simulink model "model_crmorm"  (R2012b)
settings: Solver=ode45  StartTime=0.0  StopTime=tsim  MaxStep=0.01  RelTol=1e-3
values from neighbouring files (symbols this model uses):
  am = -1    [master_crmorm.m]
  ap = 1    [master_crmorm.m]
  gamma = 100    [sim_setup.m]
  km = 1    [master_crmorm.m]
  kp = 2    [master_crmorm.m]
  l = -1000    [sim_setup.m]
  xp0 = 0    [master_crmorm.m]
settings Model: Creator=Dan  LastModifiedBy=Dan

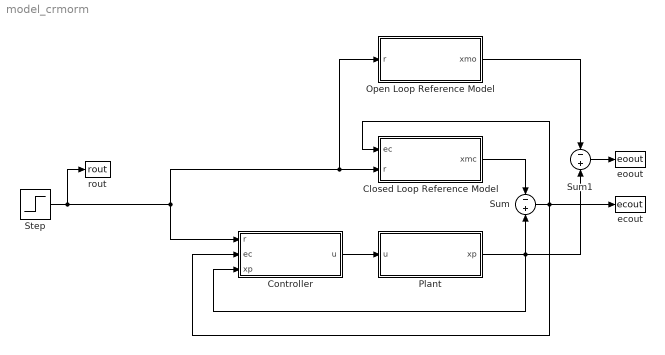
== system model_crmorm ==
  Closed Loop Reference Model : Subsystem
  Controller : Subsystem
  Open Loop Reference Model : Subsystem
  Plant : Subsystem
  Step : Step  Time=5  SampleTime=0
  Sum : Sum  Inputs=-|+
  Sum1 : Sum  Inputs=-|+
  ecout : ToWorkspace  VariableName=ecout  SampleTime=-1  SaveFormat=Structure With Time
  eoout : ToWorkspace  VariableName=eoout  SampleTime=-1  SaveFormat=Structure With Time
  rout : ToWorkspace  VariableName=rout  SampleTime=-1  SaveFormat=Structure With Time
  wires:
  Step/1 -> rout/1, Open Loop Reference Model/1(r), Closed Loop Reference Model/2(r), Controller/1(r)
  Controller/1(u) -> Plant/1(u)
  Plant/1(xp) -> Sum1/2, Sum/2, Controller/3(xp)
  Closed Loop Reference Model/1(xmc) -> Sum/1
  Sum/1 -> ecout/1, Controller/2(ec), Closed Loop Reference Model/1(ec)
  Open Loop Reference Model/1(xmo) -> Sum1/1
  Sum1/1 -> eoout/1

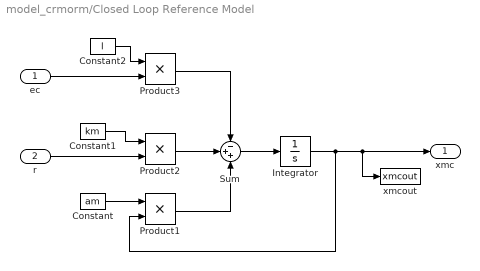
== system model_crmorm/Closed Loop Reference Model ==
  ec : Inport
  r : Inport  Port=2
  Constant : Constant  Value=am
  Constant1 : Constant  Value=km
  Constant2 : Constant  Value=l
  Integrator : Integrator
  Product1 : Product  RndMeth=Zero
  Product2 : Product  RndMeth=Zero
  Product3 : Product  RndMeth=Zero
  Sum : Sum  Inputs=-++
  xmcout : ToWorkspace  VariableName=xmcout  SampleTime=-1  SaveFormat=Structure With Time
  xmc : Outport
  wires:
  Constant/1 -> Product1/1
  Integrator/1 -> xmcout/1, xmc/1, Product1/2
  Constant1/1 -> Product2/1
  Sum/1 -> Integrator/1
  r/1 -> Product2/2
  ec/1 -> Product3/2
  Constant2/1 -> Product3/1
  Product2/1 -> Sum/2
  Product1/1 -> Sum/3
  Product3/1 -> Sum/1

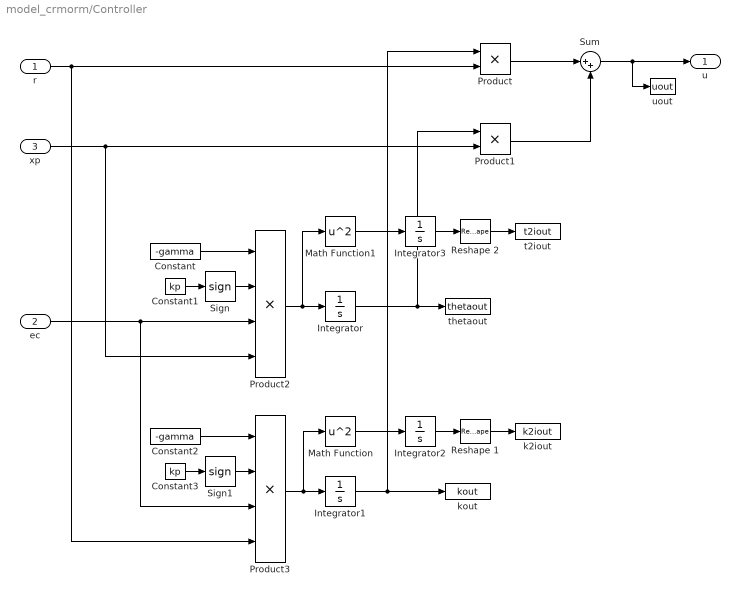
== system model_crmorm/Controller ==
  r : Inport
  ec : Inport  Port=2
  xp : Inport  Port=3
  Constant : Constant  Value=-gamma
  Constant1 : Constant  Value=kp
  Constant2 : Constant  Value=-gamma
  Constant3 : Constant  Value=kp
  Integrator{,1..3} (4 alike) : Integrator
  Math Function : Math  Operator=square  SaturateOnIntegerOverflow=on
  Math Function1 : Math  Operator=square  SaturateOnIntegerOverflow=on
  Product : Product  RndMeth=Zero
  Product1 : Product  RndMeth=Zero
  Product2 : Product  Inputs=4  RndMeth=Zero
  Product3 : Product  Inputs=4  RndMeth=Zero
  Reshape 1 : Reshape
  Reshape 2 : Reshape
  Sign : Signum
  Sign1 : Signum
  Sum : Sum  Inputs=|++
  k2iout : ToWorkspace  VariableName=k2iout  SampleTime=-1  SaveFormat=Structure With Time
  kout : ToWorkspace  VariableName=kout  SampleTime=-1  SaveFormat=Structure With Time
  t2iout : ToWorkspace  VariableName=t2iout  SampleTime=-1  SaveFormat=Structure With Time
  thetaout : ToWorkspace  VariableName=thetaout  SampleTime=-1  SaveFormat=Structure With Time
  uout : ToWorkspace  VariableName=uout  SampleTime=-1  SaveFormat=Structure With Time
  u : Outport
  wires:
  Product/1 -> Sum/1
  Product1/1 -> Sum/2
  r/1 -> Product3/4, Product/2
  xp/1 -> Product2/4, Product1/2
  Sum/1 -> uout/1, u/1
  Constant/1 -> Product2/1
  Sign/1 -> Product2/2
  Constant1/1 -> Sign/1
  Constant2/1 -> Product3/1
  Sign1/1 -> Product3/2
  Constant3/1 -> Sign1/1
  ec/1 -> Product2/3, Product3/3
  Product3/1 -> Math Function/1, Integrator1/1
  Product2/1 -> Math Function1/1, Integrator/1
  Integrator/1 -> thetaout/1, Product1/1
  Integrator1/1 -> kout/1, Product/1
  Math Function/1 -> Integrator2/1
  Math Function1/1 -> Integrator3/1
  Integrator3/1 -> Reshape 2/1
  Integrator2/1 -> Reshape 1/1
  Reshape 2/1 -> t2iout/1
  Reshape 1/1 -> k2iout/1

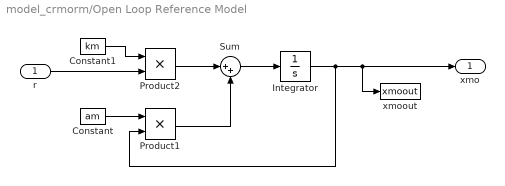
== system model_crmorm/Open Loop Reference Model ==
  r : Inport
  Constant : Constant  Value=am
  Constant1 : Constant  Value=km
  Integrator : Integrator
  Product1 : Product  RndMeth=Zero
  Product2 : Product  RndMeth=Zero
  Sum : Sum  Inputs=|++
  xmoout : ToWorkspace  VariableName=xmoout  SampleTime=-1  SaveFormat=Structure With Time
  xmo : Outport
  wires:
  Constant/1 -> Product1/1
  Integrator/1 -> xmoout/1, xmo/1, Product1/2
  Constant1/1 -> Product2/1
  Sum/1 -> Integrator/1
  r/1 -> Product2/2
  Product2/1 -> Sum/1
  Product1/1 -> Sum/2

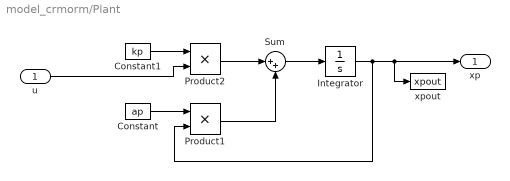
== system model_crmorm/Plant ==
  u : Inport
  Constant : Constant  Value=ap
  Constant1 : Constant  Value=kp
  Integrator : Integrator  InitialCondition=xp0
  Product1 : Product  RndMeth=Zero
  Product2 : Product  RndMeth=Zero
  Sum : Sum  Inputs=|++
  xpout : ToWorkspace  VariableName=xpout  SampleTime=-1  SaveFormat=Structure With Time
  xp : Outport
  wires:
  Constant/1 -> Product1/1
  Integrator/1 -> xpout/1, xp/1, Product1/2
  Constant1/1 -> Product2/1
  Product2/1 -> Sum/1
  Sum/1 -> Integrator/1
  Product1/1 -> Sum/2
  u/1 -> Product2/2
